simulink model "main"  (Simulink 10.0)
settings: Solver=ode3  StartTime=SimStartTime  StopTime=SimStopTime  FixedStep=0.1  RelTol=1e-3  EnableMultiTasking=on
values from neighbouring files (symbols this model uses):
  Cp =     [CpRisoe.mat]
  D = 0.4    [main.m]
  del_Plost = Pref_4567/Pbase_ps    [sub.m]
  droop = 0.04    [main.m]
  Ki = 0.2    [main.m]
  Konline = sum(online .* Pn_units) / Pbase_ps    [sub.m]
  Kp = 2    [main.m]
  Kwt2pu = Nwt / Pbase_ps    [sub.m]
  M = sum(online.*Iconv_units.*Pn_units(1:7))/Pbase_ps+2*Iwf_pu_ps    [sub.m]
  Ngear = 99.2    [main.m]
  pitch_max = 30    [main.m]
  pitch_min = 0    [main.m]
  pitch_rate_max = 10    [main.m]
  pitch_rate_min = -10    [main.m]
  Power_wt0 = 500 * 10^6    (= 500000000)    [main.m]
  R = Diam/2    (= 63)    [main.m]
  TCH = 5    [main.m]
  Ti = 2.2    [main.m]
  Tservo = 0.3    [main.m]
undefined symbols (not defined in the file or in its folder): Iechiv, MPPT_Table, omega_gen_base, omega_gen_init, omega_gen_nom, P_wt, pitch_init, rho, speed_wind, x_PI_init, x_PI_max, x_PI_min
settings Model: Creator=anca  LastModifiedBy=edxu96
settings DataIOCC: LimitDataPoints=on  SignalLoggingSaveFormat=ModelDataLogs
settings OptimizationCC: ExpressionDepthLimit=2147483647
settings DebuggingCC: SolverPrmCheckMsg=warning  FcnCallInpInsideContextMsg=warning  StateNameClashWarn=warning
settings GRTTargetCC: GeneratePreprocessorConditionals=Disable all
settings ConfigComp: CovExternalEMLEnable=off

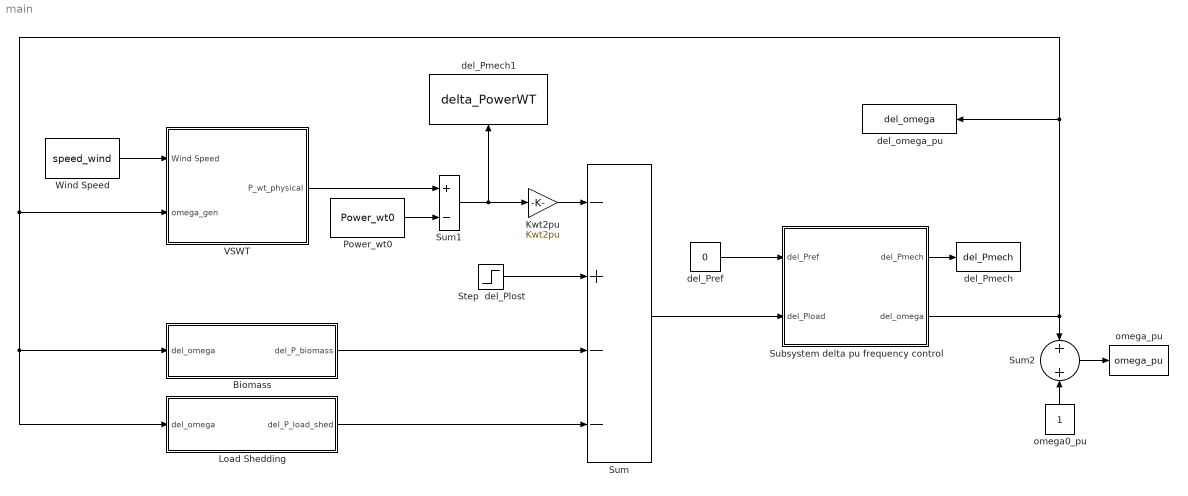
== system main ==
  "Biomass " : Subsystem  mask{fn=0, act_freq_high=0, act_freq_low=0, droop=0, TCH=0, Pnom=0, Pbase_total=0}
      mask prompts: fn "Nominal frequency [Hz]"; act_freq_high "Higher Activation Frequency [Hz]"; act_freq_low "Lower Activation Frequency [Hz]"; droop "Droop [%]"; TCH "Time constant of prime mover [s]"; Pnom "Nominal Capacity of Biomass [W]"; Pbase_total "Power System Base [W]"
  Kwt2pu : Gain  Gain=Kwt2pu
  Load Shedding : Subsystem  mask{act_freq=0, prop_PL0=0, Total_load=0, Pbase_sys=0}
      mask prompts: act_freq "Activation Frequency"; prop_PL0 "Proportion of load to be disconnected[%]"; Total_load "Total Load [W]"; Pbase_sys "Power System Base [W]"
  Power_wt0 : Constant  Value=Power_wt0
  Step  del_Plost : Step  Time=0  After=del_Plost  SampleTime=0
  Subsystem delta pu frequency control : Subsystem
  Sum : Sum  Inputs=-+--
  Sum1 : Sum  Inputs=+-
  Sum2 : Sum
  VSWT : Subsystem
  Wind Speed : Constant  Value=speed_wind
  del_Pmech : ToWorkspace  VariableName=del_Pmech  SaveFormat=Structure With Time  SampleTime=-1
  del_Pmech1 : ToWorkspace  VariableName=delta_PowerWT  SaveFormat=Structure With Time  SampleTime=-1
  del_Pref : Constant  Value=0
  del_omega_pu : ToWorkspace  VariableName=del_omega  SaveFormat=Structure With Time  SampleTime=-1
  omega0_pu : Constant
  omega_pu : ToWorkspace  VariableName=omega_pu  SaveFormat=Structure With Time  SampleTime=-1
  wires:
  del_Pref/1 -> Subsystem delta pu frequency control/1(del_Pref)
  Sum/1 -> Subsystem delta pu frequency control/2(del_Pload)
  VSWT/1(P_wt_physical) -> Sum1/1
  Power_wt0/1 -> Sum1/2
  Sum1/1 -> Kwt2pu/1, del_Pmech1/1
  Kwt2pu/1 -> Sum/1
  Step  del_Plost/1 -> Sum/2
  Subsystem delta pu frequency control/2(del_omega) -> Sum2/1, del_omega_pu/1, Load Shedding/1(del_omega), "Biomass "/1(del_omega), VSWT/2(omega_gen)
  Subsystem delta pu frequency control/1(del_Pmech) -> del_Pmech/1
  Sum2/1 -> omega_pu/1
  omega0_pu/1 -> Sum2/2
  "Biomass "/1(del_P_biomass) -> Sum/3
  Load Shedding/1(del_P_load_shed) -> Sum/4
  Wind Speed/1 -> VSWT/1(Wind Speed)

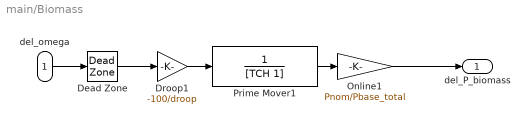
== system main/Biomass  ==
  del_omega : Inport
  Dead Zone : DeadZone  LowerValue=-(fn-act_freq_low)/fn  UpperValue=(act_freq_high-fn)/fn  SaturateOnIntegerOverflow=on
  Droop1 : Gain  Gain=-100/droop
  Online1 : Gain  Gain=Pnom/Pbase_total
  Prime Mover1 : TransferFcn  Denominator=[TCH 1]
  del_P_biomass : Outport
  wires:
  Droop1/1 -> Prime Mover1/1
  Prime Mover1/1 -> Online1/1
  Dead Zone/1 -> Droop1/1
  del_omega/1 -> Dead Zone/1
  Online1/1 -> del_P_biomass/1

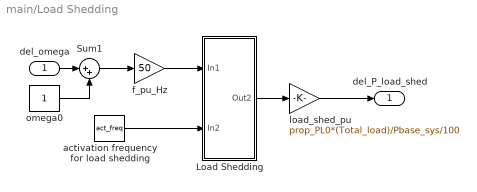
== system main/Load Shedding ==
  del_omega : Inport
  Load Shedding : Subsystem
  Sum1 : Sum  Inputs=|++
  activation frequency for load shedding : Constant  Value=act_freq
  f_pu_Hz : Gain  Gain=50
  load_shed_pu : Gain  Gain=prop_PL0*(Total_load)/Pbase_sys/100
  omega0 : Constant
  del_P_load_shed : Outport
  wires:
  Load Shedding/1(Out2) -> load_shed_pu/1
  load_shed_pu/1 -> del_P_load_shed/1
  f_pu_Hz/1 -> Load Shedding/1(In1)
  activation frequency for load shedding/1 -> Load Shedding/2(In2)
  del_omega/1 -> Sum1/1
  Sum1/1 -> f_pu_Hz/1
  omega0/1 -> Sum1/2

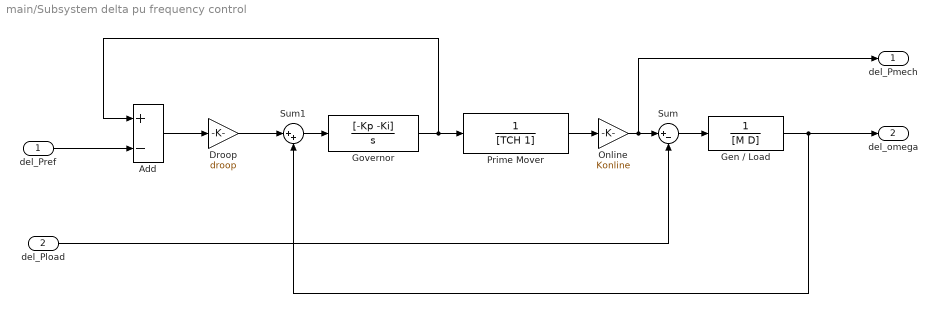
== system main/Subsystem delta pu frequency control ==
  del_Pref : Inport
  del_Pload : Inport  Port=2
  Add : Sum  Inputs=+-
  Droop : Gain  Gain=droop
  Gen / Load : TransferFcn  Denominator=[M D]
  Governor : TransferFcn  Numerator=[-Kp -Ki]  Denominator=[1 0]
  Online : Gain  Gain=Konline
  Prime Mover : TransferFcn  Denominator=[TCH 1]
  Sum : Sum  Inputs=|+-
  Sum1 : Sum  Inputs=|++
  del_Pmech : Outport
  del_omega : Outport  Port=2
  wires:
  del_Pref/1 -> Add/2
  Online/1 -> del_Pmech/1, Sum/1
  Prime Mover/1 -> Online/1
  Add/1 -> Droop/1
  Droop/1 -> Sum1/1
  Sum1/1 -> Governor/1
  Governor/1 -> Add/1, Prime Mover/1
  del_Pload/1 -> Sum/2
  Sum/1 -> Gen / Load/1
  Gen / Load/1 -> del_omega/1, Sum1/2

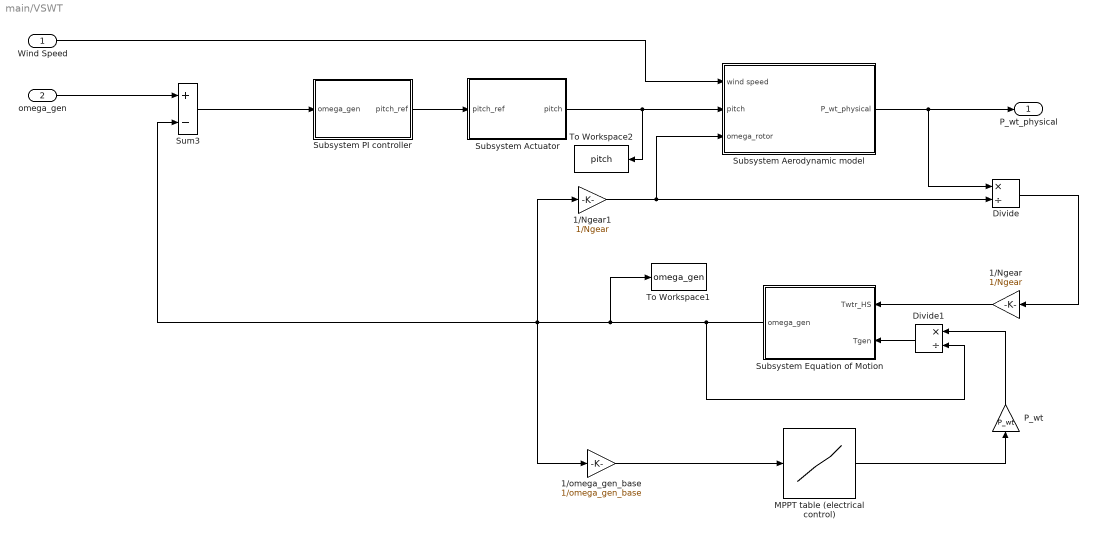
== system main/VSWT ==
  Wind Speed : Inport
  omega_gen : Inport  Port=2
  1/Ngear : Gain  Gain=1/Ngear
  1/Ngear1 : Gain  Gain=1/Ngear
  1/omega_gen_base : Gain  Gain=1/omega_gen_base
  Divide : Product  Inputs=*/
  Divide1 : Product  Inputs=*/
  MPPT table (electrical control) : Lookup_n-D  NumberOfTableDimensions=1  BreakpointsForDimension1=MPPT_Table(1,:)  Table=MPPT_Table(2,:)  RndMeth=Simplest  InputSameDT=on
  P_wt : Gain  Gain=P_wt
  Subsystem Actuator : Subsystem
  Subsystem Aerodynamic model : Subsystem
  Subsystem Equation of Motion : Subsystem
  Subsystem PI controller : Subsystem
  Sum3 : Sum  Inputs=+-
  To Workspace1 : ToWorkspace  VariableName=omega_gen  SaveFormat=Structure With Time  SampleTime=-1
  To Workspace2 : ToWorkspace  VariableName=pitch  SaveFormat=Structure With Time  SampleTime=-1
  P_wt_physical : Outport
  wires:
  omega_gen/1 -> Sum3/1
  Sum3/1 -> Subsystem PI controller/1(omega_gen)
  MPPT table (electrical control)/1 -> P_wt/1
  Divide1/1 -> Subsystem Equation of Motion/2(Tgen)
  1/omega_gen_base/1 -> MPPT table (electrical control)/1
  1/Ngear/1 -> Subsystem Equation of Motion/1(Twtr_HS)
  Subsystem Actuator/1(pitch) -> Subsystem Aerodynamic model/2(pitch), To Workspace2/1
  P_wt/1 -> Divide1/1
  Subsystem PI controller/1(pitch_ref) -> Subsystem Actuator/1(pitch_ref)
  1/Ngear1/1 -> Subsystem Aerodynamic model/3(omega_rotor), Divide/2
  Divide/1 -> 1/Ngear/1
  Subsystem Aerodynamic model/1(P_wt_physical) -> P_wt_physical/1, Divide/1
  Subsystem Equation of Motion/1(omega_gen) -> Divide1/2, Sum3/2, 1/Ngear1/1, 1/omega_gen_base/1, To Workspace1/1
  Wind Speed/1 -> Subsystem Aerodynamic model/1(wind speed)

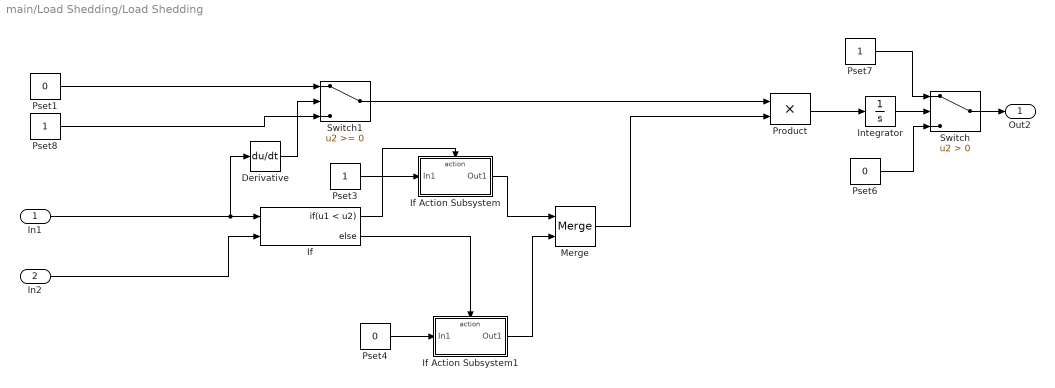
== system main/Load Shedding/Load Shedding ==
  In1 : Inport
  In2 : Inport  Port=2
  Derivative : Derivative  CoefficientInTFapproximation=0
  If : If  NumInputs=2  IfExpression=u1 < u2
  If Action Subsystem : Subsystem  TreatAsAtomicUnit=on
  If Action Subsystem1 : Subsystem  TreatAsAtomicUnit=on
  Integrator : Integrator
  Merge : Merge
  Product : Product
  Pset1 : Constant  Value=0
  Pset3 : Constant
  Pset4 : Constant  Value=0
  Pset6 : Constant  Value=0
  Pset7 : Constant
  Pset8 : Constant
  Switch : Switch  Criteria=u2 > Threshold
  Switch1 : Switch  ZeroCross=off
  Out2 : Outport
  wires:
  If Action Subsystem/1(Out1) -> Merge/1
  If Action Subsystem1/1(Out1) -> Merge/2
  Pset6/1 -> Switch/3
  Switch/1 -> Out2/1
  Integrator/1 -> Switch/2
  Pset7/1 -> Switch/1
  Merge/1 -> Product/2
  Pset8/1 -> Switch1/3
  Pset1/1 -> Switch1/1
  In2/1 -> If/2
  If/2 -> If Action Subsystem1/Action
  Pset4/1 -> If Action Subsystem1/1(In1)
  In1/1 -> If/1, Derivative/1
  Pset3/1 -> If Action Subsystem/1(In1)
  If/1 -> If Action Subsystem/Action
  Product/1 -> Integrator/1
  Switch1/1 -> Product/1
  Derivative/1 -> Switch1/2

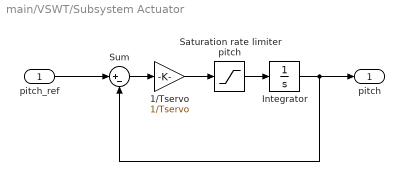
== system main/VSWT/Subsystem Actuator ==
  pitch_ref : Inport
  1/Tservo : Gain  Gain=1/Tservo
  Integrator : Integrator  InitialCondition=pitch_init  LimitOutput=on  UpperSaturationLimit=pitch_max  LowerSaturationLimit=pitch_min
  Saturation rate limiter pitch : Saturate  UpperLimit=pitch_rate_max  LowerLimit=pitch_rate_min
  Sum : Sum  Inputs=|+-
  pitch : Outport
  wires:
  1/Tservo/1 -> Saturation rate limiter pitch/1
  Sum/1 -> 1/Tservo/1
  Saturation rate limiter pitch/1 -> Integrator/1
  pitch_ref/1 -> Sum/1
  Integrator/1 -> pitch/1, Sum/2

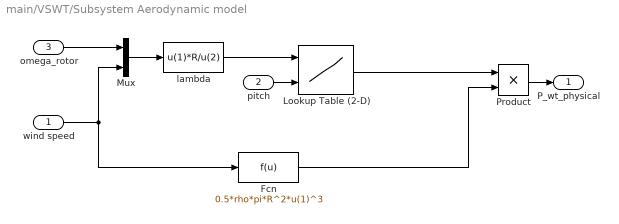
== system main/VSWT/Subsystem Aerodynamic model ==
  wind speed : Inport
  pitch : Inport  Port=2
  omega_rotor : Inport  Port=3
  Fcn : Fcn  Expr=0.5*rho*pi*R^2*u(1)^3
  Lookup Table (2-D) : Lookup2D  RowIndex=Cp.lambda  ColumnIndex=Cp.pitch  Table=Cp.values
  Mux : Mux  Inputs=2
  Product : Product  RndMeth=Zero
  lambda : Fcn  Expr=u(1)*R/u(2)
  P_wt_physical : Outport
  wires:
  Product/1 -> P_wt_physical/1
  pitch/1 -> Lookup Table (2-D)/2
  omega_rotor/1 -> Mux/1
  Fcn/1 -> Product/2
  Lookup Table (2-D)/1 -> Product/1
  lambda/1 -> Lookup Table (2-D)/1
  Mux/1 -> lambda/1
  wind speed/1 -> Fcn/1, Mux/2

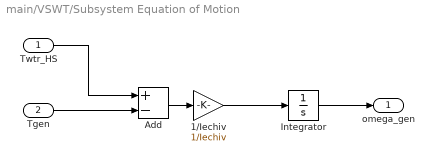
== system main/VSWT/Subsystem Equation of Motion ==
  Twtr_HS : Inport
  Tgen : Inport  Port=2
  1/Iechiv : Gain  Gain=1/Iechiv
  Add : Sum  Inputs=+-
  Integrator : Integrator  InitialCondition=omega_gen_init
  omega_gen : Outport
  wires:
  Integrator/1 -> omega_gen/1
  1/Iechiv/1 -> Integrator/1
  Add/1 -> 1/Iechiv/1
  Twtr_HS/1 -> Add/1
  Tgen/1 -> Add/2

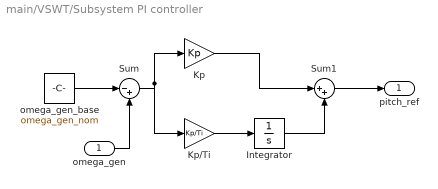
== system main/VSWT/Subsystem PI controller ==
  omega_gen : Inport
  Integrator : Integrator  InitialCondition=x_PI_init  LimitOutput=on  UpperSaturationLimit=x_PI_max  LowerSaturationLimit=x_PI_min
  Kp : Gain  Gain=Kp
  Kp/Ti : Gain  Gain=Kp/Ti
  Sum : Sum  Inputs=|-+
  Sum1 : Sum  Inputs=|++
  omega_gen_base : Constant  Value=omega_gen_nom
  pitch_ref : Outport
  wires:
  omega_gen/1 -> Sum/2
  omega_gen_base/1 -> Sum/1
  Sum/1 -> Kp/1, Kp/Ti/1
  Kp/Ti/1 -> Integrator/1
  Kp/1 -> Sum1/1
  Integrator/1 -> Sum1/2
  Sum1/1 -> pitch_ref/1

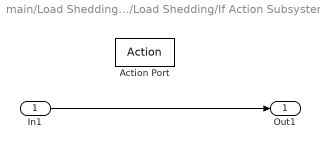
== system main/Load Shedding/Load Shedding/If Action Subsystem ==
  In1 : Inport
  Action Port : ActionPort
  Out1 : Outport
  wires:
  In1/1 -> Out1/1

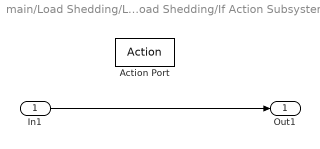
== system main/Load Shedding/Load Shedding/If Action Subsystem1 ==
  In1 : Inport
  Action Port : ActionPort
  Out1 : Outport
  wires:
  In1/1 -> Out1/1
